simulink model "modelocarro"  (R2017a)
settings: Solver=VariableStepAuto  StartTime=0.0  StopTime=10.0  RelTol=1e-3
values from neighbouring files (symbols this model uses):
  Beqtran = (0 + Beqrot/(Rr^2))    (= 120)    [datoscarro.m]
  Meq = (mc + Jeq/(Rr^2))    (= 59008)    [datoscarro.m]
  Rr = 0.5    [datoscarro.m]
  rt = 15.0    (= 15)    [datoscarro.m]
settings Model: Creator=tomas  LastModifiedBy=tomas

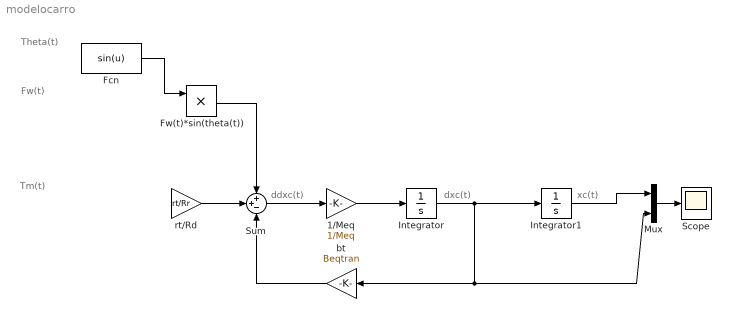
== system modelocarro ==
  note: Tm(t)
  note: Fw(t)
  note: Theta(t)
  note: ddxc(t)
  note: xc(t)
  note: dxc(t)
  1/Meq : Gain  Gain=1/Meq
  Fcn : Fcn  Expr=sin(u)
  Fw(t)*sin(theta(t)) : Product
  Integrator : Integrator
  Integrator1 : Integrator
  Mux : Mux  Inputs=2
  Scope : Scope
  Sum : Sum  Inputs=++-
  bt : Gain  Gain=Beqtran
  rt/Rd : Gain  Gain=rt/Rr
  wires:
  Sum/1 -> 1/Meq/1
  1/Meq/1 -> Integrator/1
  Integrator/1 -> Mux/2, bt/1, Integrator1/1
  Fw(t)*sin(theta(t))/1 -> Sum/1
  rt/Rd/1 -> Sum/2
  ? -> rt/Rd/1
  bt/1 -> Sum/3
  Integrator1/1 -> Mux/1
  ? -> Fw(t)*sin(theta(t))/2
  Fcn/1 -> Fw(t)*sin(theta(t))/1
  ? -> Fcn/1
  Mux/1 -> Scope/1
